simulink library "adcscope_lib"  (Simulink 6.2)
libraries: xbsIndex_r3 x36, xps_library x7, adcscope_lib x2
settings Model: LastModifiedBy=hchen05

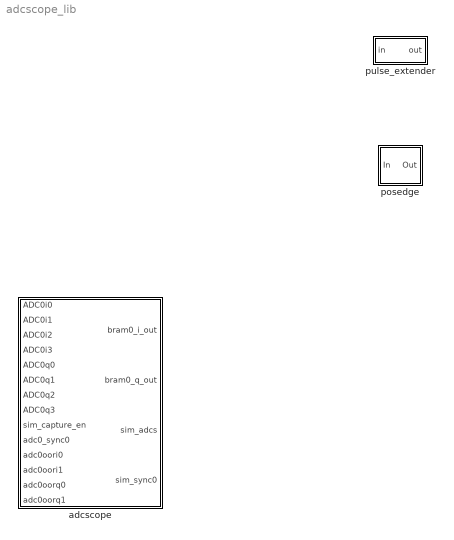
== system adcscope_lib ==
  adcscope : Subsystem  mask{num_adcs=1, interleave=on, address_width=11}
      mask prompts: num_adcs "Number of ADCs"; interleave "Interleave mode (set your ADCs accordingly)"; address_width "BRAM address width (2^?)"
      mask init:
      | adcscope_mask;
      mask StyleString: popup(1|2),checkbox,edit
  posedge : Subsystem  Tag=Rising Edge Detector  mask{yummy=on}
      mask prompts: yummy "Cookies are great!"
  pulse_extender : Subsystem  mask{pulse_len=2^12-1}
      mask prompts: pulse_len "Length of Pulse"
      mask init:
      | bits = ceil(log2(pulse_len));

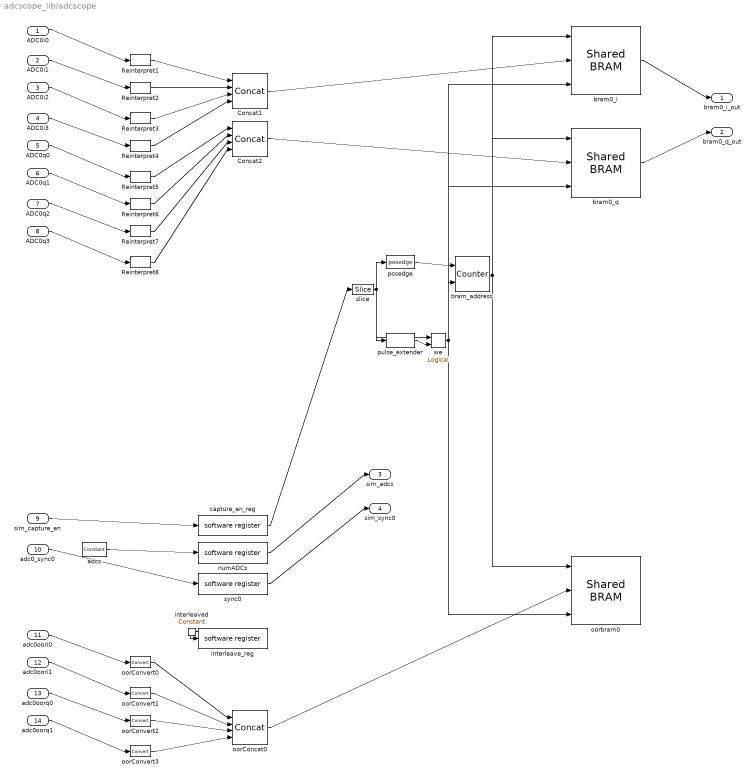
== system adcscope_lib/adcscope ==
  ADC0i0 : Inport  Port=1  LatchInput=off
  ADC0i1 : Inport  Port=2  LatchInput=off
  ADC0i2 : Inport  Port=3  LatchInput=off
  ADC0i3 : Inport  Port=4  LatchInput=off
  ADC0q0 : Inport  Port=5  LatchInput=off
  ADC0q1 : Inport  Port=6  LatchInput=off
  ADC0q2 : Inport  Port=7  LatchInput=off
  ADC0q3 : Inport  Port=8  LatchInput=off
  sim_capture_en : Inport  Port=9  LatchInput=off
  adc0_sync0 : Inport  Port=10  LatchInput=off
  adc0oori0 : Inport  Port=11  LatchInput=off
  adc0oori1 : Inport  Port=12  LatchInput=off
  adc0oorq0 : Inport  Port=13  LatchInput=off
  adc0oorq1 : Inport  Port=14  LatchInput=off
  Concat1 : xbsIndex_r3/Concat  num_inputs=4  explicit_period=off  period=1  dbl_ovrd=off
  Concat2 : xbsIndex_r3/Concat  num_inputs=4  explicit_period=off  period=1  dbl_ovrd=off
  Reinterpret{1..8} (8 alike) : xbsIndex_r3/Reinterpret  force_arith_type=on  arith_type=Unsigned  force_bin_pt=on  bin_pt=0  force_valid=on
  adcs : xbsIndex_r3/Constant  const=1  equ=P=C  arith_type=Unsigned  n_bits=1  bin_pt=0  opselect=C  inp2=PCIN>>17  opr=+  inp1=P  carry=CIN  iostate=0  explicit_period=on  period=1  dbl_ovrd=off
  bram0_i : xps_library/Shared BRAM  Tag=xps:bram  arith_type=Unsigned  addr_width=address_width  data_width=32  data_bin_pt=0  init_vals=zeros(1, 2^address_width)  sample_rate=1
  bram0_q : xps_library/Shared BRAM  Tag=xps:bram  arith_type=Unsigned  addr_width=address_width  data_width=32  data_bin_pt=0  init_vals=zeros(1, 2^address_width)  sample_rate=1
  bram_address : xbsIndex_r3/Counter  cnt_type=Free Running  n_bits=address_width  bin_pt=0  arith_type=Unsigned  start_count=0  cnt_to=Inf  cnt_by_val=1  operation=Up  explicit_period=off  period=1  load_pin=off  rst=on  en=on  dbl_ovrd=off  show_param=off  use_rpm=on  gen_core=off
      settings: xl_area=[0, 0, 0, 0, 0, 0, 0]
  capture_en_reg : xps_library/software register  Tag=xps:sw_reg  io_dir=From Processor  arith_type=Unsigned  bitwidth=32  bin_pt=0  sample_period=1  gw_name=adcscope_lib_adcscope_capture_en_reg_user_data_out
  interleave_reg : xps_library/software register  Tag=xps:sw_reg  io_dir=To Processor  arith_type=Unsigned  bitwidth=32  bin_pt=0  sample_period=1  gw_name=adcscope_lib_adcscope_interleave_reg_user_data_in
  interleaved : xbsIndex_r3/Constant  const=1  equ=P=C  arith_type=Unsigned  n_bits=1  bin_pt=0  opselect=C  inp2=PCIN>>17  opr=+  inp1=P  carry=CIN  iostate=0  explicit_period=on  period=1  dbl_ovrd=off
  numADCs : xps_library/software register  Tag=xps:sw_reg  io_dir=To Processor  arith_type=Unsigned  bitwidth=32  bin_pt=0  sample_period=1  gw_name=adcscope_lib_adcscope_numADCs_user_data_in
  oorConcat0 : xbsIndex_r3/Concat  num_inputs=4  explicit_period=off  period=1  dbl_ovrd=off
  oorConvert{0..3} (4 alike) : xbsIndex_r3/Convert  arith_type=Unsigned  n_bits=8  bin_pt=0  quantization=Truncate  overflow=Wrap  latency=0  explicit_period=off  period=1  dbl_ovrd=off  show_param=off  inserted_by_tool=off  pipeline=off
      settings: xl_area=[0, 0, 0, 0, 0, 0, 0]
  oorbram0 : xps_library/Shared BRAM  Tag=xps:bram  arith_type=Unsigned  addr_width=address_width  data_width=32  data_bin_pt=0  init_vals=zeros(1, 2^address_width)  sample_rate=1
  posedge : adcscope_lib/posedge  Tag=Rising Edge Detector  yummy=on
  pulse_extender : adcscope_lib/pulse_extender  pulse_len=2^address_width-1
  slice : xbsIndex_r3/Slice  mode=Lower Bit Location + Width  nbits=1  bit1=0  base1=MSB of Input  bit0=0  base0=LSB of Input  boolean_output=on  explicit_period=off  period=1  dbl_ovrd=off
  sync0 : xps_library/software register  Tag=xps:sw_reg  io_dir=To Processor  arith_type=Unsigned  bitwidth=32  bin_pt=0  sample_period=1  gw_name=adcscope_lib_adcscope_sync0_user_data_in
  we : xbsIndex_r3/Logical  logical_function=AND  inputs=2  precision=Full  arith_type=Unsigned  n_bits=8  bin_pt=2  align_bp=on  latency=0  explicit_period=off  period=1  en=off  dbl_ovrd=off  show_param=off
      settings: xl_area=[0, 0, 0, 0, 0, 0, 0]
  bram0_i_out : Outport
  bram0_q_out : Outport  Port=2
  sim_adcs : Outport  Port=3
  sim_sync0 : Outport  Port=4
  wires:
  sim_capture_en/1 -> capture_en_reg/1
  capture_en_reg/1 -> slice/1
  adc0_sync0/1 -> sync0/1
  sync0/1 -> sim_sync0/1
  adcs/1 -> numADCs/1
  numADCs/1 -> sim_adcs/1
  interleaved/1 -> interleave_reg/1
  ADC0q3/1 -> Reinterpret8/1
  ADC0q2/1 -> Reinterpret7/1
  ADC0q1/1 -> Reinterpret6/1
  ADC0q0/1 -> Reinterpret5/1
  ADC0i3/1 -> Reinterpret4/1
  ADC0i2/1 -> Reinterpret3/1
  ADC0i1/1 -> Reinterpret2/1
  ADC0i0/1 -> Reinterpret1/1
  Reinterpret8/1 -> Concat2/4
  Reinterpret7/1 -> Concat2/3
  Reinterpret6/1 -> Concat2/2
  Reinterpret5/1 -> Concat2/1
  Reinterpret4/1 -> Concat1/4
  Reinterpret3/1 -> Concat1/3
  Reinterpret2/1 -> Concat1/2
  Reinterpret1/1 -> Concat1/1
  Concat1/1 -> bram0_i/2
  Concat2/1 -> bram0_q/2
  bram0_i/1 -> bram0_i_out/1
  bram0_q/1 -> bram0_q_out/1
  bram_address/1 -> bram0_i/1, bram0_q/1, oorbram0/1
  posedge/1 -> bram_address/1
  pulse_extender/1 -> we/2
  slice/1 -> we/1, posedge/1, pulse_extender/1
  we/1 -> bram_address/2, bram0_i/3, bram0_q/3, oorbram0/3
  adc0oori0/1 -> oorConvert0/1
  adc0oori1/1 -> oorConvert1/1
  adc0oorq0/1 -> oorConvert2/1
  adc0oorq1/1 -> oorConvert3/1
  oorConvert3/1 -> oorConcat0/4
  oorConvert2/1 -> oorConcat0/3
  oorConvert1/1 -> oorConcat0/2
  oorConvert0/1 -> oorConcat0/1
  oorConcat0/1 -> oorbram0/2

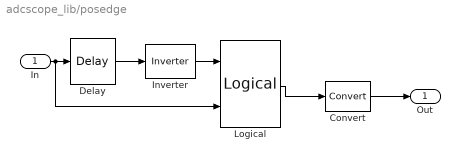
== system adcscope_lib/posedge ==
  In : Inport  Port=1  LatchInput=off
  Convert : xbsIndex_r3/Convert  arith_type=Boolean  n_bits=8  bin_pt=6  quantization=Truncate  overflow=Wrap  latency=0  explicit_period=off  period=1  dbl_ovrd=off  show_param=off  inserted_by_tool=off  pipeline=off
      settings: xl_area=[0, 0, 0, 0, 0, 0, 0]
  Delay : xbsIndex_r3/Delay  latency=1  reg_retiming=off  explicit_period=off  period=1  en=off  accept_only_valid=off  init_zero=on  dbl_ovrd=off  show_param=off
      settings: xl_area=[0, 0, 0, 0, 0, 0, 0]
  Inverter : xbsIndex_r3/Inverter  latency=0  explicit_period=off  period=1  en=off  dbl_ovrd=off  show_param=off
      settings: xl_area=[0, 0, 0, 0, 0, 0, 0]
  Logical : xbsIndex_r3/Logical  logical_function=AND  inputs=2  precision=Full  arith_type=Unsigned  n_bits=8  bin_pt=2  align_bp=on  latency=0  explicit_period=off  period=1  en=off  dbl_ovrd=off  show_param=off
      settings: xl_area=[0, 0, 0, 0, 0, 0, 0]
  Out : Outport
  wires:
  Logical/1 -> Convert/1
  In/1 -> Logical/2, Delay/1
  Inverter/1 -> Logical/1
  Delay/1 -> Inverter/1
  Convert/1 -> Out/1

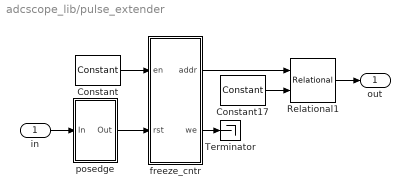
== system adcscope_lib/pulse_extender ==
  in : Inport  Port=1  LatchInput=off
  Constant : xbsIndex_r3/Constant  const=1  equ=P=C  arith_type=Boolean  n_bits=1  bin_pt=0  opselect=C  inp2=PCIN>>17  opr=+  inp1=P  carry=CIN  iostate=0  explicit_period=on  period=1  dbl_ovrd=off
  Constant17 : xbsIndex_r3/Constant  const=pulse_len  equ=P=C  arith_type=Unsigned  n_bits=bits  bin_pt=0  opselect=C  inp2=PCIN>>17  opr=+  inp1=P  carry=CIN  iostate=0  explicit_period=on  period=1  dbl_ovrd=off
  Relational1 : xbsIndex_r3/Relational  mode=a<b  latency=0  explicit_period=off  period=1  en=off  dbl_ovrd=off  show_param=off
      settings: xl_area=[0, 0, 0, 0, 0, 0, 0]
  Terminator : Terminator
  freeze_cntr : Subsystem  mask{CounterBits=bits}
      mask prompts: CounterBits "Counter Length (2^?)"
  posedge : Subsystem  Tag=Rising Edge Detector
  out : Outport
  wires:
  Constant/1 -> freeze_cntr/1(en)
  freeze_cntr/2(we) -> Terminator/1
  freeze_cntr/1(addr) -> Relational1/1
  posedge/1(Out) -> freeze_cntr/2(rst)
  Constant17/1 -> Relational1/2
  Relational1/1 -> out/1
  in/1 -> posedge/1(In)

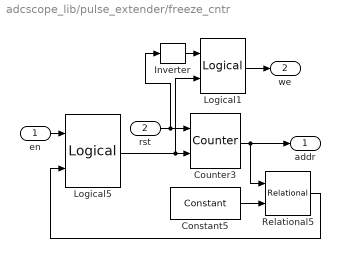
== system adcscope_lib/pulse_extender/freeze_cntr ==
  en : Inport  Port=1  LatchInput=off
  rst : Inport  Port=2  LatchInput=off
  Constant5 : xbsIndex_r3/Constant  const=2^CounterBits - 1  equ=P=C  arith_type=Unsigned  n_bits=CounterBits  bin_pt=0  opselect=C  inp2=PCIN>>17  opr=+  inp1=P  carry=CIN  iostate=0  explicit_period=on  period=1  dbl_ovrd=off
  Counter3 : xbsIndex_r3/Counter  cnt_type=Free Running  n_bits=CounterBits  bin_pt=0  arith_type=Unsigned  start_count=0  cnt_to=1023  cnt_by_val=1  operation=Up  explicit_period=on  period=1  load_pin=off  rst=on  en=on  dbl_ovrd=off  show_param=off  use_rpm=on  gen_core=off
      settings: xl_area=[0, 0, 0, 0, 0, 0, 0]
  Inverter : xbsIndex_r3/Inverter  latency=0  explicit_period=off  period=1  en=off  dbl_ovrd=off  show_param=off
      settings: xl_area=[0, 0, 0, 0, 0, 0, 0]
  Logical1 : xbsIndex_r3/Logical  logical_function=AND  inputs=2  precision=Full  arith_type=Unsigned  n_bits=8  bin_pt=2  align_bp=on  latency=0  explicit_period=off  period=1  en=off  dbl_ovrd=off  show_param=off
      settings: xl_area=[0, 0, 0, 0, 0, 0, 0]
  Logical5 : xbsIndex_r3/Logical  logical_function=AND  inputs=2  precision=Full  arith_type=Unsigned  n_bits=8  bin_pt=2  align_bp=on  latency=0  explicit_period=off  period=1  en=off  dbl_ovrd=off  show_param=off
      settings: xl_area=[0, 0, 0, 0, 0, 0, 0]
  Relational5 : xbsIndex_r3/Relational  mode=a!=b  latency=0  explicit_period=off  period=1  en=off  dbl_ovrd=off  show_param=off
      settings: xl_area=[0, 0, 0, 0, 0, 0, 0]
  addr : Outport
  we : Outport  Port=2
  wires:
  rst/1 -> Counter3/1, Inverter/1
  Logical5/1 -> Counter3/2, Logical1/2
  en/1 -> Logical5/1
  Relational5/1 -> Logical5/2
  Constant5/1 -> Relational5/2
  Counter3/1 -> Relational5/1, addr/1
  Inverter/1 -> Logical1/1
  Logical1/1 -> we/1

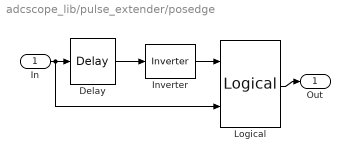
== system adcscope_lib/pulse_extender/posedge ==
  In : Inport  Port=1  LatchInput=off
  Delay : xbsIndex_r3/Delay  latency=1  reg_retiming=off  explicit_period=off  period=1  en=off  accept_only_valid=off  init_zero=on  dbl_ovrd=off  show_param=off
      settings: xl_area=[0, 0, 0, 0, 0, 0, 0]
  Inverter : xbsIndex_r3/Inverter  latency=0  explicit_period=off  period=1  en=off  dbl_ovrd=off  show_param=off
      settings: xl_area=[0, 0, 0, 0, 0, 0, 0]
  Logical : xbsIndex_r3/Logical  logical_function=AND  inputs=2  precision=Full  arith_type=Unsigned  n_bits=8  bin_pt=2  align_bp=on  latency=0  explicit_period=off  period=1  en=off  dbl_ovrd=off  show_param=off
      settings: xl_area=[0, 0, 0, 0, 0, 0, 0]
  Out : Outport
  wires:
  Delay/1 -> Inverter/1
  Inverter/1 -> Logical/1
  In/1 -> Delay/1, Logical/2
  Logical/1 -> Out/1
